simulink model "power_wind_dfig_avg"  (R2022b)
settings: Solver=ode113  StartTime=0.0  StopTime=200  RelTol=1e-3
PreLoadFcn:
  | Ts=5e-6;
InitFcn:
  | %load myModel_init;
  | Ts=5e-5;
undefined symbols (not defined in the file or in its folder): D1, D11, Delta, DiscIntNeverNeededParam, find_system
libraries: powerlib_extras x72, simulink x18, eeSinusoidalMeasurement x17, simulink_extras x12, spsThreePhaseVIMeasurementLib x11, spsControlledVoltageSourceLib x8, spsThreePhaseTransformerTwoWindingsLib x5, spsThreePhasePISectionLineLib x2, spsAsynchronousMachinepuUnitsLib x2, spsThreePhaseSeriesRLCBranchLib x2, spsThreePhaseSeriesRLCLoadLib x2, spsGroundLib x2
(part 2 of 6)

== system power_wind_dfig_avg/Wind Farm ==
  note: 9 MW Wind Farm
      | (6 x 1.5 MW)
  25 kV/ 575 V 6*1.75MVA : spsThreePhaseTransformerTwoWindingsLib/Three-Phase Transformer (Two Windings)  Winding1Connection=Delta (D11)  Winding2Connection=Yg  CoreType=Three single-phase transformers  SetSaturation=off  Hysteresis=off  DataFile='hysteresis'  SetInitialFlux=off  Measurements=None  UNITS=pu  NominalPower="[1.75e6*NoT  60]"  Winding1=[25e3 , 1e-6 0.15]  Winding2=[ 575, 1e-6 0]  Rm=500  Lm=500  L0=0.5  Saturation=[ 0,0 ; 0.0024,1.2 ; 1.0,1.52 ]  InitialFluxes=[ 0.8 , -0.8 , 0.7 ]  BreakLoop=off  DiscreteSolver=Trapezoidal iterative  DataType=off  TransfoNumber=0
  30 km line : spsThreePhasePISectionLineLib/Three-Phase PI Section Line  LConnTagsString=a|b|c  RConnTagsString=A|B|C  Length=30  Frequency=60  Resistances=[0.1153 0.413]  Inductances=[1.05e-3 3.32e-3]  Capacitances=[11.33e-009 5.01e-009]
  B25 : spsThreePhaseVIMeasurementLib/Three-Phase V-I Measurement  VoltageMeasurement=phase-to-ground  SetLabelV=off  LabelV=Vabc_B230  Vpu=on  VpuLL=off  CurrentMeasurement=yes  SetLabelI=off  LabelI=Iabc_B230  Ipu=on  Pbase=NoT*1.5e6/0.9  Vbase=25e3  OutputType=Complex  PhasorSimulation=off  PSBequivalent=0
  B575 (575 V) : spsThreePhaseVIMeasurementLib/Three-Phase V-I Measurement  VoltageMeasurement=phase-to-ground  SetLabelV=off  LabelV=Vabc_B575  Vpu=on  VpuLL=off  CurrentMeasurement=yes  SetLabelI=off  LabelI=Iabc_B575  Ipu=on  Pbase=NoT*1.5e6/0.9  Vbase=575  OutputType=Complex  PhasorSimulation=off  PSBequivalent=0
  Bus Creator : BusCreator  Inputs=5
  Bus Creator1 : BusCreator  Inputs=2
  Bus Selector1 : BusSelector  OutputSignals=Vdc_V,wr_pu (IG speed),PQ_pu.P_pu,PQ_pu.Q_pu
  Bus Selector2 : BusSelector  OutputSignals=Magnitude_sig.phiqrA,Magnitude_sig.phidrA,Magnitude_sig.iqsA,Magnitude_sig.idsA,Magnitude_sig.VqrA,Magnitude_sig.VdrA,m.Mechanical.Rotor speed (wm),m.Mechanical.Electromagnetic torque Te (pu),m.Rotor measurements.Rotor flux phir_q (pu),m.Rotor measurements.Rotor flux phir_d (pu),m.Stator measurements.Stator flux phis_q (pu),m.Stator measurements.Stator flux phis_d (pu)  OutputAsBus=on
  Constant : Constant  Value=TurOn
  Constant2 : Constant  Value=11
  Constant3 : Constant  Value=0
  DFIG Wind Turbine : Subsystem  LoadFcn=%find_system(gcs,'FollowLinks', 'on', 'LookUnderMasks', 'all');  mask(DFIG Wind Turbine){Nb_wt=NoT, ShowParameters=Generator data for 1 wind turbine, nom=[1.5e6/.9 575 1975 60], sta=[ 0.023 0.18], rot=[ 0.016 0.16], Lm=2.9, mec=[0.685 0.01 3], init=[ -0.2,0   0,0,0   0,0,0 ], Imax_grid_conv=0.8, RL_grid=[ 0.3 0.003], Vdc_nom=1150, C_DClink1=10000e-6, C_var_filter1=120e3, Pmec1=1.5e6, wind_speed_CpMax=11, wind0=11, DisplayTurbChar=off, H_WT=4.32, Ksh=1.11, D_mutual=1.5, w_wt0=1.2, torque0=0.83, Kdc=[8   400], Kgrid_side_cur_reg=[0.83 5], Kspeed=[3 0.6], Krotor_side_cur_reg=[0.6 8], Ki_QV=[0.05 20], Kp_pitch=[150], Kcompensation=[3 30], pitch_max=27, pitch_rate=0}
      mask prompts: Nb_wt "Number of wind turbines:"; ShowParameters "Display:"; nom "Nom. power, L-L volt. and freq. [Pn (VA), Vs_nom (Vrms), Vr_nom (Vrms), fn (Hz)]:"; sta "Stator [ Rs,Lls ] (p.u.):"; rot "Rotor [ Rr',Llr' ] (p.u.):"; Lm "Magnetizing inductance Lm (p.u.):"; mec "Inertia constant, friction factor, and pairs of poles [ H(s)  F(p.u.)  p ]:"; init "Initial conditions [s  th  ias  ibs  ics  phaseas phasebs phasecs]:"; Imax_grid_conv "Grid-side converter maximum current (pu of generator nominal current):"; RL_grid "Grid-side coupling inductor [ L, R] (p.u.):"; Vdc_nom "Nominal DC bus voltage (V):"; C_DClink1 "DC bus capacitor (F):"; C_var_filter1 "Line filter capacitor (Q=50) (var):"; Pmec1 "Nominal mechanical output power (W):"; wind_speed_CpMax "Wind speed at nominal speed and at Cp max (must be between 6 m/s and 30 m/s) (m/s):"; wind0 "Initial wind speed (m/s):"; DisplayTurbChar "Display wind turbine power characteristics:"; H_WT "Wind turbine inertia constant H (s):"; Ksh "Shaft spring constant refer to high-speed shaft (pu of nominal mechanical torque/rad):"; D_mutual "Shaft mutual damping (pu of nominal mechanical torque/pu dw):"; w_wt0 "Turbine initial speed (pu of nominal speed):"; torque0 "Initial output torque (pu of nominal mechanical torque):"; Kdc "DC bus voltage regulator gains [Kp Ki]:"; Kgrid_side_cur_reg "Grid-side converter current regulator gains [Kp Ki]:"; Kspeed "Speed regulator gains [Kp Ki]:"; Krotor_side_cur_reg "Rotor-side converter current regulator gains [Kp Ki]:"; Ki_QV "Q and V regulator gains [Ki_var Ki_volt]:"; Kp_pitch "Pitch controller gain [Kp]:"; Kcompensation "Pitch compensation gains [Kp Ki]:"; pitch_max "Maximum pitch angle (deg):"; pitch_rate "Maximum rate of change of pitch angle (deg/s):"
      mask help: This block implements a model of a variable speed pitch controlled wind turbine using a doubly-fed induction generator (DFIG).
      mask init: same as power_wind_dfig_avg/DFIG Wind Turbine
      mask TypeOptions ShowParameters: Generator data for 1 wind turbine | Converters data for 1 wind turbine | Turbine data for 1 wind turbine | Drive train data for 1 wind turbine | Control parameters for 1 wind turbine
      mask Callback ShowParameters:
      | BlockName=getfullname(gcb);
      | %
      | Param_Show=get_param(BlockName,'ShowParameters');
      | Param_DisplayTurbChar=get_param(BlockName,'DisplayTurbChar');
      | 
      | p_mask{3}='off';p_mask{4}='off';p_mask{5}='off';
      | p_mask{6}='off';p_mask{7}='off';p_mask{8}='off';p_mask{9}='off';
      | p_mask{10}='off';p_mask{11}='off';p_mask{12}='off';p_mask{13}='off';
      | p_mask{14}='off';p_mask{15}='off';p_mask{16}='off';p_mask{17}='off';
      | p_mask{18}='off';p_mask{19}='off';p_mask{20}='off';p_mask{21}='off';
      | p_mask{22}='off';p_mask{23}='off';p_mask{24}='off';p_mask{25}='off';
      | p_mask{26}='off';p_mask{27}='off';p_mask{28}='off';p_mask{29}='off';
      | p_mask{30}='off';p_mask{31}='off';
      | 
      | 
      | switch Param_Show
      | 	case 'Generator data for 1 wind turbine'
      | 		p_mask{3}='on';p_mask{4}='on';p_mask{5}='on'; p_mask{6}='on';
      |         p_mask{7}='on'; p_mask{8}='on';
      |     case 'Converters data for 1 wind turbine'
      | 		p_mask{9}='on';p_mask{10}='on';p_mask{11}='on';p_mask{12}='on';
      |         p_mask{13}='on';
      | 	case 'Turbine data for 1 wind turbine'
      |         p_mask{14}='on';p_mask{15}='on';p_mask{16}='on';p_mask{17}='on';
      |     case 'Drive train data for 1 wind turbine'
      |         p_mask{18}='on';p_mask{19}='on';p_mask{20}='on';p_mask{21}='on';
      |         p_mask{22}='on';
      |     case 'Control parameters for 1 wind turbine'
      |         p_mask{23}='on';p_mask{24}='on';p_mask{25}='on';
      |         p_mask{26}='on';p_mask{27}='on';p_mask{28}='on';p_mask{29}='on';
      |         p_mask{30}='on'; p_mask{31}='on';
      | end
      | 
      | ParVisible={'on','on',p_mask{3},p_mask{4},p_mask{5},p_mask{6},p_mask{7},...
      |     p_mask{8},p_mask{9},p_mask{10},p_mask{11},p_mask{12},p_mask{13},...
      |     p_mask{14},p_mask{15},p_mask{16},p_mask{17},p_mask{18},p_mask{19},...
      |     p_mask{20},p_mask{21},p_mask{22},p_mask{23},p_mask{24},p_mask{25},...
      |     p_mask{26},p_mask{27},p_mask{28},p_mask{29},p_mask{30},p_mask{31},...
      |     };
      | %
      | set_param(BlockName,'MaskVisibilities',ParVisible);
      | set_param(BlockName,'DisplayTurbChar',Param_DisplayTurbChar);
  Demux : Demux  Commented=on  Outputs=2
  From10 : From  Commented=on  GotoTag=Q_pu
      settings: CloseFcn=tagdialog Close
  From11 : From  Commented=on  GotoTag=P_pu
      settings: CloseFcn=tagdialog Close
  From3 : From  Commented=on  GotoTag=Vabc_B230
      settings: CloseFcn=tagdialog Close
  From4 : From  Commented=on  GotoTag=Iabc_B230
      settings: CloseFcn=tagdialog Close
  From6 : From  Commented=on  GotoTag=Vdc
      settings: CloseFcn=tagdialog Close
  From7 : From  Commented=on  GotoTag=wr
      settings: CloseFcn=tagdialog Close
  From8 : From  Commented=on  GotoTag=Vabc_B575
      settings: CloseFcn=tagdialog Close
  From9 : From  Commented=on  GotoTag=Iabc_B575
      settings: CloseFcn=tagdialog Close
  MW : Gain  Commented=on  Gain=NoT*1.5/0.9  SaturateOnIntegerOverflow=on  OutDataTypeStr=Inherit: Same as input  ParamDataTypeStr=Inherit: Same as input
  Manual Switch : ManualSwitch  CurrentSetting=0
  Mux : Mux  Commented=on  Inputs=2
  "Power (3ph, Instantaneous)" : spsPower3phInstantaneousLib/Power (3ph, Instantaneous)
  Product : Product  Inputs=3
  Scope : Scope  Commented=on  NumInputPorts=8
  Sine Wave Function : Sin  Amplitude=Ampl  Frequency=2*pi*Freq  Phase=0/4*pi  SampleTime=0
  Step : Step  Time=Stept  SampleTime=0
  Sum : Sum  Inputs=|+-
  Sum1 : Sum  Inputs=++|
  Terminator : Terminator
  Terminator1 : Terminator
  Three-Phase Sinusoidal Measurement (PLL) : eeSinusoidalMeasurement/Sinusoidal Measurement (PLL, Three-Phase)  Kp_LF=200  Ki_LF=2000  F0=60  Theta0=0  Ts=-1
  Three-Phase Sinusoidal Measurement (PLL)1 : eeSinusoidalMeasurement/Sinusoidal Measurement (PLL, Three-Phase)  Kp_LF=200  Ki_LF=2000  F0=60  Theta0=0  Ts=-1
  To Workspace : ToWorkspace  VariableName=windspeed  SaveFormat=Timeseries  SampleTime=-1
  wind speed m : Subsystem
  A : PMIOPort  Side=Left
  B : PMIOPort  Port=2  Side=Left
  C : PMIOPort  Port=3  Side=Left
  Macsig : Outport  VectorParamsAs1DForOutWhenUnconnected=off
  Gridsig : Outport  Port=2  VectorParamsAs1DForOutWhenUnconnected=off
  wires:
  [Vabc_B575] -> Three-Phase Sinusoidal Measurement (PLL)/1
  [Vabc_B575] -> "Power (3ph, Instantaneous)"/1
  Three-Phase Sinusoidal Measurement (PLL)/1 -> Terminator/1
  Constant3/1 -> DFIG Wind Turbine/2(Qref_pu)
  Constant2/1 -> Sum1/2
  Bus Selector1/3 -> [P_pu]  "<P_pu>"
  From3/1 -> Scope/7  "Vabc_B25 (pu)"
  Bus Creator/1 -> Gridsig/1
  Three-Phase Sinusoidal Measurement (PLL)1/2 -> Sum/2
  Demux/2 -> Scope/4  "Q (Mvar)"
  From9/1 -> Scope/2  "Iabc_B575 (pu)"
  From6/1 -> Scope/5  "Vdc (V)"
  Mux/1 -> MW/1
  Demux/1 -> Scope/3  "P (MW)"
  From4/1 -> Scope/8  "Iabc_B25 (pu)"
  [Iabc_B575] -> "Power (3ph, Instantaneous)"/2
  Bus Selector1/2 -> wind speed m/1(rotor speed), [wr]  "<wr_pu (IG speed)>"
  [Vabc_B230] -> Three-Phase Sinusoidal Measurement (PLL)1/1
  Step/1 -> Product/1
  Product/1 -> Sum1/1
  From7/1 -> Scope/6  "wr (pu)"
  Three-Phase Sinusoidal Measurement (PLL)/3 -> Bus Creator/4  "Vi"
  Bus Selector1/4 -> [Q_pu]  "<Q_pu>"
  Three-Phase Sinusoidal Measurement (PLL)1/3 -> Bus Creator/5  "Vj"
  Sine Wave Function/1 -> Product/2
  "Power (3ph, Instantaneous)"/1 -> Bus Creator/1  "SourceP"
  DFIG Wind Turbine/1(m) -> Bus Selector1/1
  From8/1 -> Scope/1  "Vabc_B575 (pu)"
  Three-Phase Sinusoidal Measurement (PLL)/2 -> Sum/1  "Thetai"
  "Power (3ph, Instantaneous)"/2 -> Bus Creator/2  "SourceQ"
  Sum/1 -> Bus Creator/3  "Thetaij"
  MW/1 -> Demux/1
  Bus Selector1/1 -> [Vdc]  "<Vdc_V>"
  From11/1 -> Mux/1
  From10/1 -> Mux/2
  Three-Phase Sinusoidal Measurement (PLL)1/1 -> Terminator1/1
  Constant/1 -> Product/3
  DFIG Wind Turbine/2(Magnitude_sig) -> Bus Creator1/1
  DFIG Wind Turbine/3(Macmeasure) -> Bus Creator1/2
  Bus Creator1/1 -> Bus Selector2/1
  Bus Selector2/1 -> Macsig/1
  B575 (575 V)/2 -> [Iabc_B575]
  B575 (575 V)/1 -> [Vabc_B575]
  B25/1 -> [Vabc_B230]
  B25/2 -> [Iabc_B230]
  wind speed m/1(wind speed) -> Manual Switch/1, To Workspace/1
  Sum1/1 -> Manual Switch/2
  Manual Switch/1 -> DFIG Wind Turbine/1("Wind (m/s) ")
  connections:
  B575 (575 V)/RConn3 -- DFIG Wind Turbine/LConn3
  B25/RConn3 -- 30 km line/LConn3
  25 kV/ 575 V 6*1.75MVA/RConn3 -- B575 (575 V)/LConn3
  B25/LConn1 -- A/RConn1
  30 km line/RConn2 -- 25 kV/ 575 V 6*1.75MVA/LConn2
  25 kV/ 575 V 6*1.75MVA/RConn2 -- B575 (575 V)/LConn2
  30 km line/RConn1 -- 25 kV/ 575 V 6*1.75MVA/LConn1
  30 km line/RConn3 -- 25 kV/ 575 V 6*1.75MVA/LConn3
  B575 (575 V)/RConn1 -- DFIG Wind Turbine/LConn1
  B25/RConn2 -- 30 km line/LConn2
  25 kV/ 575 V 6*1.75MVA/RConn1 -- B575 (575 V)/LConn1
  B575 (575 V)/RConn2 -- DFIG Wind Turbine/LConn2
  B25/RConn1 -- 30 km line/LConn1
  B25/LConn2 -- B/RConn1
  B25/LConn3 -- C/RConn1

== system power_wind_dfig_avg/info ==

== system power_wind_dfig_avg/wind speed m ==
  rotor speed : Inport
  Add : Sum
  Add1 : Sum
  Add2 : Sum
  Band-Limited White Noise : simulink/Sources/Band-Limited White Noise  Cov=[5]  Ts=0.1  seed=[34242]
  Band-Limited White Noise1 : simulink/Sources/Band-Limited White Noise  Cov=[5]  Ts=0.1  seed=[31141]
  Band-Limited White Noise2 : simulink/Sources/Band-Limited White Noise  Cov=[5]  Ts=0.1  seed=[32053]
  Cosine : simulink/Lookup Tables/Cosine  Commented=on  Formula=cos(2*pi*u)  NumDataPoints=(2^5)+1  OutputWordLength=16  InternalRulePriority=Speed
  Delay : Delay  Commented=on  DelayLength=1  InitialCondition=0
  Delay1 : Delay  Commented=on  DelayLength=1  InitialCondition=0
  Gain : Gain  Commented=on  Gain=3
  Gain1 : Gain  Commented=on  Gain=sqrt(2)
  Gain2 : Gain  Commented=on  Gain=sqrt(2)
  Gain3 : Gain  Commented=on  Gain=2*pi
  Integrator : Integrator  Commented=on  WrapState=on  WrappedStateUpperValue=2*pi  WrappedStateLowerValue=0
  Product : Product
  Product1 : Product
  Scope : Scope
  Sine : simulink/Lookup Tables/Sine  Commented=on  Formula=sin(2*pi*u)  NumDataPoints=(2^5)+1  OutputWordLength=16  InternalRulePriority=Speed
  Transfer Fcn : TransferFcn  Numerator=[4.7869 0.9904]  Denominator=[7.6823 7.3518 1]
  Transfer Fcn1 : TransferFcn  Numerator=[0.2766 0.0307]  Denominator=[0.3691 1.7722 1]
  Transfer Fcn2 : TransferFcn  Numerator=[0.2766 0.0307]  Denominator=[0.3691 1.7722 1]
  Transfer Fcn3 : TransferFcn  Numerator=[0.0182 1.3653 0.9846]  Denominator=[1.3463 3.7593 1]
  Transfer Fcn4 : TransferFcn  Numerator=[0.0182 1.3653 0.9846]  Denominator=[1.3463 3.7593 1]
  Transfer Fcn5 : TransferFcn  Numerator=[0.0182 1.3653 0.9846]  Denominator=[1.3463 3.7593 1]
  average wind speed : Constant  Value=11
  wind speed : Outport  VectorParamsAs1DForOutWhenUnconnected=off
  wires:
  average wind speed/1 -> Add/1
  Transfer Fcn/1 -> Add/2
  Delay1/1 -> Product1/1
  Gain1/1 -> Delay/1
  Transfer Fcn5/1 -> Transfer Fcn2/1
  Add2/1 -> wind speed/1, Scope/1
  Add/1 -> Add2/1
  Band-Limited White Noise2/1 -> Transfer Fcn5/1
  Delay/1 -> Product/2
  Cosine/1 -> Gain2/1
  Product/1 -> Add1/1
  Add1/1 -> Add2/2
  Gain2/1 -> Delay1/1
  Transfer Fcn3/1 -> Transfer Fcn1/1
  Band-Limited White Noise1/1 -> Transfer Fcn3/1
  Transfer Fcn2/1 -> Product1/2
  Product1/1 -> Add1/2
  Gain/1 -> Cosine/1, Sine/1
  Sine/1 -> Gain1/1
  Band-Limited White Noise/1 -> Transfer Fcn4/1
  Transfer Fcn4/1 -> Transfer Fcn/1
  Transfer Fcn1/1 -> Product/1
  Integrator/1 -> Gain/1
  rotor speed/1 -> Gain3/1
  Gain3/1 -> Integrator/1

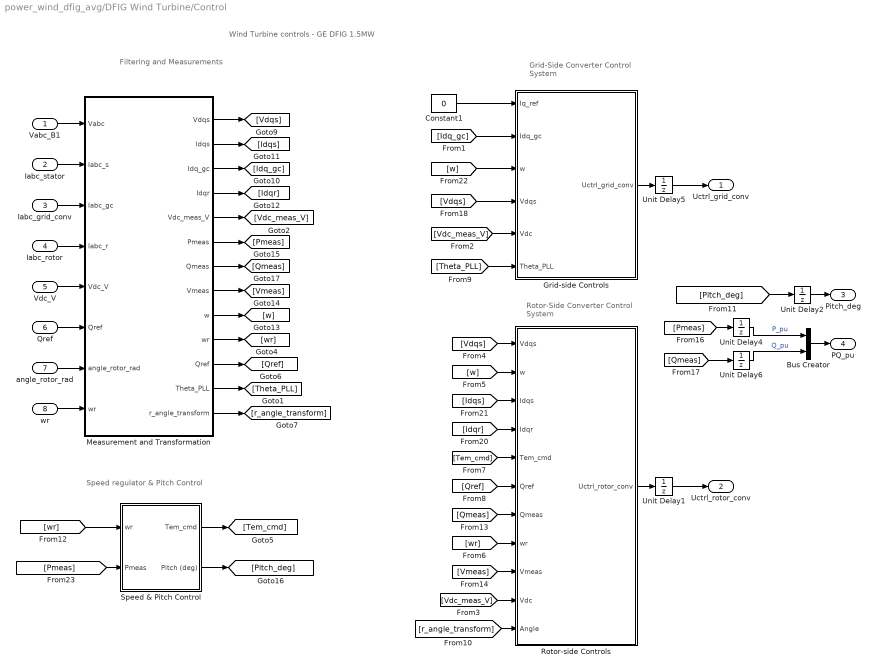
== system power_wind_dfig_avg/DFIG Wind Turbine/Control ==
  note: Speed regulator & Pitch Control
  note: Grid-Side Converter
      | Control System
  note: Rotor-Side Converter
      | Control System
  note: Filtering and
      | Measurements
  note: Wind Turbine controls - GE DFIG 1.5MW
  Vabc_B1 : Inport
  Iabc_stator : Inport  Port=2
  Iabc_grid_conv : Inport  Port=3
  Iabc_rotor : Inport  Port=4
  Vdc_V : Inport  Port=5
  Qref : Inport  Port=6
  angle_rotor_rad : Inport  Port=7
  wr : Inport  Port=8
  Bus Creator : BusCreator  Inputs=2
  Constant1 : Constant  Value=0
  Grid-side Controls : Subsystem
  Measurement and Transformation : Subsystem
  Rotor-side Controls : Subsystem
  Speed & Pitch Control : Subsystem
  Unit Delay{1..2,4..6} (5 alike) : UnitDelay  SampleTime=Ts  HasFrameUpgradeWarning=on
  Uctrl_grid_conv : Outport  VectorParamsAs1DForOutWhenUnconnected=off
  Uctrl_rotor_conv : Outport  Port=2  VectorParamsAs1DForOutWhenUnconnected=off
  Pitch_deg : Outport  Port=3  VectorParamsAs1DForOutWhenUnconnected=off
  PQ_pu : Outport  Port=4  VectorParamsAs1DForOutWhenUnconnected=off
  wires:
  Unit Delay6/1 -> Bus Creator/2  "Q_pu"
  Unit Delay4/1 -> Bus Creator/1  "P_pu"
  [Qmeas] -> Unit Delay6/1
  [Pmeas] -> Unit Delay4/1
  Bus Creator/1 -> PQ_pu/1
  Unit Delay2/1 -> Pitch_deg/1
  Unit Delay1/1 -> Uctrl_rotor_conv/1
  Unit Delay5/1 -> Uctrl_grid_conv/1
  Speed & Pitch Control/1(Tem_cmd) -> [Tem_cmd]
  Speed & Pitch Control/2(Pitch (deg)) -> [Pitch_deg]
  Rotor-side Controls/1(Uctrl_rotor_conv) -> Unit Delay1/1
  [r_angle_transform] -> Rotor-side Controls/11(Angle)
  [Vdc_meas_V] -> Rotor-side Controls/10(Vdc)
  Measurement and Transformation/13(r_angle_transform) -> [r_angle_transform]
  Grid-side Controls/1(Uctrl_grid_conv) -> Unit Delay5/1
  [Theta_PLL] -> Grid-side Controls/6(Theta_PLL)
  Measurement and Transformation/12(Theta_PLL) -> [Theta_PLL]
  [Vmeas] -> Rotor-side Controls/9(Vmeas)
  Measurement and Transformation/8(Vmeas) -> [Vmeas]
  [Qmeas] -> Rotor-side Controls/7(Qmeas)
  Measurement and Transformation/7(Qmeas) -> [Qmeas]
  Vabc_B1/1 -> Measurement and Transformation/1(Vabc)
  Iabc_grid_conv/1 -> Measurement and Transformation/3(Iabc_gc)
  Iabc_rotor/1 -> Measurement and Transformation/4(Iabc_r)
  Iabc_stator/1 -> Measurement and Transformation/2(Iabc_s)
  angle_rotor_rad/1 -> Measurement and Transformation/7(angle_rotor_rad)
  Constant1/1 -> Grid-side Controls/1(Iq_ref)
  Measurement and Transformation/1(Vdqs) -> [Vdqs]
  Measurement and Transformation/2(Idqs) -> [Idqs]
  Measurement and Transformation/3(Idq_gc) -> [Idq_gc]
  Measurement and Transformation/4(Idqr) -> [Idqr]
  Measurement and Transformation/6(Pmeas) -> [Pmeas]
  Measurement and Transformation/9(w) -> [w]
  [Idq_gc] -> Grid-side Controls/2(Idq_gc)
  [w] -> Grid-side Controls/3(w)
  [Vdqs] -> Grid-side Controls/4(Vdqs)
  [Vdc_meas_V] -> Grid-side Controls/5(Vdc)
  [Vdqs] -> Rotor-side Controls/1(Vdqs)
  [w] -> Rotor-side Controls/2(w)
  [Idqs] -> Rotor-side Controls/3(Idqs)
  [Idqr] -> Rotor-side Controls/4(Idqr)
  [Tem_cmd] -> Rotor-side Controls/5(Tem_cmd)
  [Qref] -> Rotor-side Controls/6(Qref)
  [wr] -> Speed & Pitch Control/1(wr)
  Measurement and Transformation/5(Vdc_meas_V) -> [Vdc_meas_V]
  Measurement and Transformation/10("wr ") -> [wr]
  Measurement and Transformation/11("Qref ") -> [Qref]
  Vdc_V/1 -> Measurement and Transformation/5(Vdc_V)
  Qref/1 -> Measurement and Transformation/6(Qref)
  wr/1 -> Measurement and Transformation/8(wr)
  [Pmeas] -> Speed & Pitch Control/2(Pmeas)
  [Pitch_deg] -> Unit Delay2/1
  [wr] -> Rotor-side Controls/8(wr)

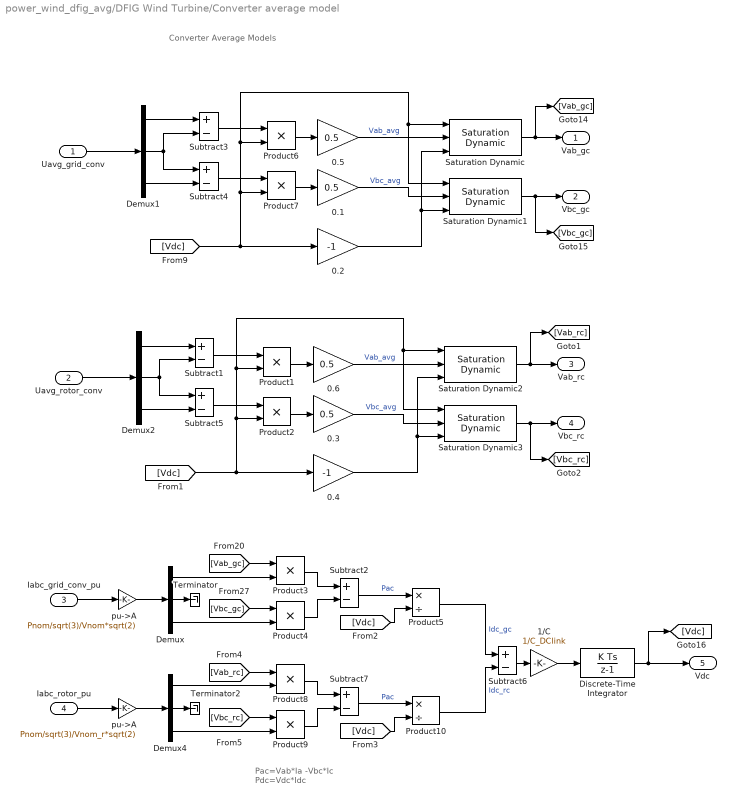
== system power_wind_dfig_avg/DFIG Wind Turbine/Converter average model ==
  note: Converter Average Models
  note: Pac=Vab*Ia -Vbc*Ic
      | Pdc=Vdc*Idc
  Uavg_grid_conv : Inport
  Uavg_rotor_conv : Inport  Port=2
  Iabc_grid_conv_pu : Inport  Port=3
  Iabc_rotor_pu : Inport  Port=4
  " pu->A" : Gain  Gain=Pnom/sqrt(3)/Vnom_r*sqrt(2)  SaturateOnIntegerOverflow=on  OutDataTypeStr=Inherit: Same as input  ParamDataTypeStr=Inherit: Same as input
  0.{1,3,5..6} (4 alike) : Gain  Gain=0.5
  0.2 : Gain  Gain=-1
  0.4 : Gain  Gain=-1
  1/C : Gain  Gain=1/C_DClink
  Demux{,1..2,4} (4 alike) : Demux  Outputs=3
  Discrete-Time Integrator : DiscreteIntegrator  InitialCondition=Vdc_nom  SampleTime=Ts  LimitOutput=on  LowerSaturationLimit=1e-6  ICPrevOutput=DiscIntNeverNeededParam  ICPrevScaledInput=DiscIntNeverNeededParam
  Product{1..4,6..9} (8 alike) : Product  RndMeth=Zero
  Product10 : Product  Inputs=*/  RndMeth=Zero
  Product5 : Product  Inputs=*/  RndMeth=Zero
  Saturation Dynamic{,1..3} (4 alike) : simulink/Discontinuities/Saturation Dynamic  OutMin=[]  OutMax=[]  OutDataTypeStr=Inherit: Same as second input  OutDataType=sfix(16)  OutScaling=2^-10  DoSatur=off
  Subtract{1..7} (7 alike) : Sum  Inputs=+-
  Terminator : Terminator
  Terminator2 : Terminator
  "pu->A " : Gain  Gain=Pnom/sqrt(3)/Vnom*sqrt(2)  SaturateOnIntegerOverflow=on  OutDataTypeStr=Inherit: Same as input  ParamDataTypeStr=Inherit: Same as input
  Vab_gc : Outport  VectorParamsAs1DForOutWhenUnconnected=off
  Vbc_gc : Outport  Port=2  VectorParamsAs1DForOutWhenUnconnected=off
  Vab_rc : Outport  Port=3  VectorParamsAs1DForOutWhenUnconnected=off
  Vbc_rc : Outport  Port=4  VectorParamsAs1DForOutWhenUnconnected=off
  Vdc : Outport  Port=5  VectorParamsAs1DForOutWhenUnconnected=off
  wires:
  " pu->A"/1 -> Demux4/1
  Demux4/2 -> Terminator2/1
  Demux4/1 -> Product8/2
  Demux4/3 -> Product9/2
  [Vdc] -> Product10/2
  [Vbc_rc] -> Product9/1
  [Vab_rc] -> Product8/1
  Product9/1 -> Subtract7/2
  Product8/1 -> Subtract7/1
  Subtract7/1 -> Product10/1  "Pac"
  Product10/1 -> Subtract6/2  "Idc_rc"
  Iabc_grid_conv_pu/1 -> "pu->A "/1
  Demux/2 -> Terminator/1
  Demux/1 -> Product3/2
  Demux/3 -> Product4/2
  Iabc_rotor_pu/1 -> " pu->A"/1
  "pu->A "/1 -> Demux/1
  Subtract6/1 -> 1/C/1
  1/C/1 -> Discrete-Time Integrator/1
  Discrete-Time Integrator/1 -> [Vdc], Vdc/1
  [Vdc] -> Product5/2
  Uavg_rotor_conv/1 -> Demux2/1
  Subtract5/1 -> Product2/1
  Subtract1/1 -> Product1/1
  Product2/1 -> 0.3/1
  Product1/1 -> 0.6/1
  Demux2/3 -> Subtract5/2
  Demux2/2 -> Subtract5/1, Subtract1/2
  Demux2/1 -> Subtract1/1
  0.6/1 -> Saturation Dynamic2/2  "Vab_avg"
  0.3/1 -> Saturation Dynamic3/2  "Vbc_avg"
  0.4/1 -> Saturation Dynamic3/3, Saturation Dynamic2/3
  Saturation Dynamic2/1 -> Vab_rc/1, [Vab_rc]
  Saturation Dynamic3/1 -> Vbc_rc/1, [Vbc_rc]
  [Vdc] -> Product2/2, Product1/2, Saturation Dynamic2/1, Saturation Dynamic3/1, 0.4/1
  Uavg_grid_conv/1 -> Demux1/1
  Subtract4/1 -> Product7/1
  Subtract3/1 -> Product6/1
  Product7/1 -> 0.1/1
  Product6/1 -> 0.5/1
  Demux1/3 -> Subtract4/2
  Demux1/2 -> Subtract3/2, Subtract4/1
  Demux1/1 -> Subtract3/1
  0.5/1 -> Saturation Dynamic/2  "Vab_avg"
  0.1/1 -> Saturation Dynamic1/2  "Vbc_avg"
  0.2/1 -> Saturation Dynamic/3, Saturation Dynamic1/3
  Saturation Dynamic/1 -> [Vab_gc], Vab_gc/1
  Saturation Dynamic1/1 -> [Vbc_gc], Vbc_gc/1
  [Vbc_gc] -> Product4/1
  [Vab_gc] -> Product3/1
  Product4/1 -> Subtract2/2
  Product3/1 -> Subtract2/1
  [Vdc] -> 0.2/1, Saturation Dynamic1/1, Saturation Dynamic/1, Product6/2, Product7/2
  Subtract2/1 -> Product5/1  "Pac"
  Product5/1 -> Subtract6/1  "Idc_gc"

== system power_wind_dfig_avg/DFIG Wind Turbine/Drive Train ==
  note: Shaft
  note: Turbine
  note: Wind turbine drive train based on a 2-masse model
  T_wt (pu) : Inport
  Generator speed (pu) : Inport  Port=2
  1_2H_WT : Gain  Gain=1/(2*H_WT)  SaturateOnIntegerOverflow=on  OutDataTypeStr=Inherit: Same as input  ParamDataTypeStr=Inherit: Same as input
  Discrete-Time Integrator : DiscreteIntegrator  InitialCondition=w_wt0  SampleTime=Ts  ICPrevOutput=DiscIntNeverNeededParam  ICPrevScaledInput=DiscIntNeverNeededParam
  Discrete-Time Integrator1 : DiscreteIntegrator  InitialCondition=torque0/Ksh  SampleTime=Ts  ICPrevOutput=DiscIntNeverNeededParam  ICPrevScaledInput=DiscIntNeverNeededParam
  Mutual damping : Gain  Gain=D_mutual  SaturateOnIntegerOverflow=on  OutDataTypeStr=Inherit: Same as input  ParamDataTypeStr=Inherit: Same as input
  Stiffness : Gain  Gain=Ksh  SaturateOnIntegerOverflow=on  OutDataTypeStr=Inherit: Same as input  ParamDataTypeStr=Inherit: Same as input
  Sum : Sum  Inputs=+-  InputSameDT=on  SaturateOnIntegerOverflow=on  OutDataTypeStr=Inherit: Same as first input
  Sum1 : Sum  Inputs=+-  InputSameDT=on  SaturateOnIntegerOverflow=on  OutDataTypeStr=Inherit: Same as first input
  Sum2 : Sum  InputSameDT=on  SaturateOnIntegerOverflow=on  OutDataTypeStr=Inherit: Same as first input
  wbase : Gain  Gain=wbase  SaturateOnIntegerOverflow=on  OutDataTypeStr=Inherit: Same as input  ParamDataTypeStr=Inherit: Same as input
  W_wt (pu) : Outport  VectorParamsAs1DForOutWhenUnconnected=off
  T_shaft (pu) : Outport  Port=2  VectorParamsAs1DForOutWhenUnconnected=off
  wires:
  wbase/1 -> Discrete-Time Integrator1/1
  Discrete-Time Integrator1/1 -> Stiffness/1
  Stiffness/1 -> Sum2/1
  Sum/1 -> 1_2H_WT/1
  1_2H_WT/1 -> Discrete-Time Integrator/1
  Discrete-Time Integrator/1 -> Sum1/1, W_wt (pu)/1
  Generator speed (pu)/1 -> Sum1/2
  Sum1/1 -> wbase/1, Mutual damping/1
  Mutual damping/1 -> Sum2/2
  Sum2/1 -> Sum/2, T_shaft (pu)/1
  T_wt (pu)/1 -> Sum/1

== system power_wind_dfig_avg/DFIG Wind Turbine/Wind Turbine ==
  W_wt (pu) : Inport
  Pitch angle (deg) : Inport  Port=2
  Wind speed (m/s) : Inport  Port=3
  ->pu : Gain  Gain=1/Prated
  Avoid div. by zero : Saturate  UpperLimit=inf  LowerLimit=eps
  "Avoid div. by zero " : Saturate  UpperLimit=inf  LowerLimit=eps
  Fcn1 : Fcn  Expr=K1*u[2]/u[1]
  Fcn2 : Fcn  Expr=c1*(c6*u[1] + (-c4 - c3*(2.5 + u[2]) + c2*(1/(u[1] + c7*(2.5 + u[2])) -c8/(1 + (2.5 + u[2])^3)))/exp(c5*(1/(u[1] + c7*(2.5 + u[2])) - c8/(1 + (2.5 + u[2])^3))))
  "K2*Cp*wind^3 " : Fcn  Expr=K2*u[1]^3*u[2]
  Mux : Mux  Inputs=2
  Mux1 : Mux  Inputs=2
  Mux2 : Mux  Inputs=2
  Product2 : Product  Inputs=*/  InputSameDT=on  SaturateOnIntegerOverflow=on  OutDataTypeStr=Inherit: Same as first input
  Tt (pu) : Outport  VectorParamsAs1DForOutWhenUnconnected=off
  wires:
  "K2*Cp*wind^3 "/1 -> ->pu/1
  "Avoid div. by zero "/1 -> Product2/2, Mux/2
  Avoid div. by zero/1 -> Mux/1, Mux2/1
  W_wt (pu)/1 -> "Avoid div. by zero "/1
  Pitch angle (deg)/1 -> Mux1/2
  Mux2/1 -> "K2*Cp*wind^3 "/1
  Fcn2/1 -> Mux2/2  "Cp"
  Mux/1 -> Fcn1/1
  Mux1/1 -> Fcn2/1
  Fcn1/1 -> Mux1/1  "lambda"
  Wind speed (m/s)/1 -> Avoid div. by zero/1
  Product2/1 -> Tt (pu)/1
  ->pu/1 -> Product2/1  "power_pu"

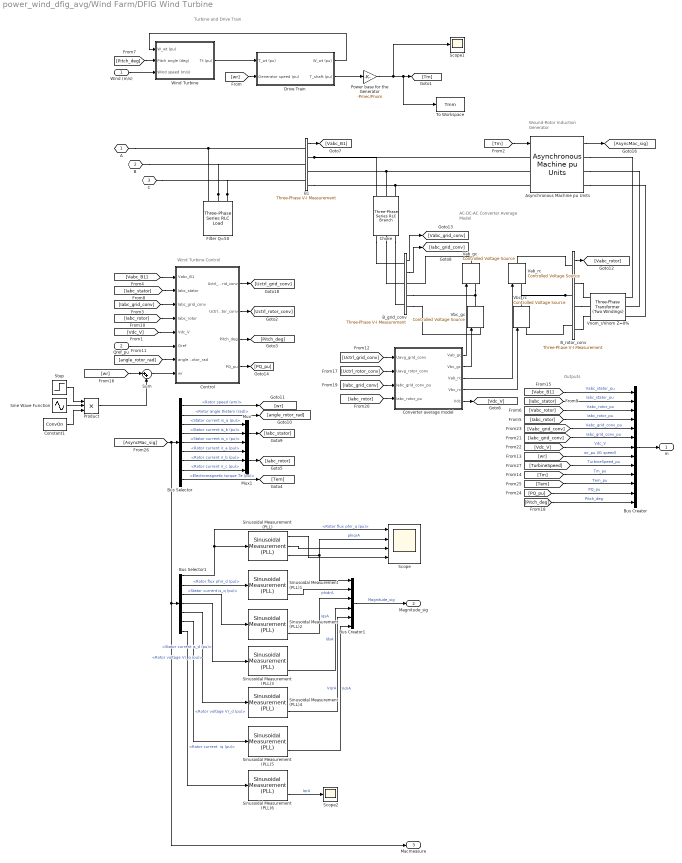
== system power_wind_dfig_avg/Wind Farm/DFIG Wind Turbine ==
  note: Turbine and Drive Train
  note: Wind Turbine Control
  note: Wound-Rotor
      | Induction Generator
  note: AC-DC-AC Converter
      | Average Model
  note: Outputs
  "Wind (m/s) " : Inport
  Qref_pu : Inport  Port=2
  Asynchronous Machine pu Units : spsAsynchronousMachinepuUnitsLib/Asynchronous Machine pu Units  RotorType=Wound  PresetModel=No  MechanicalLoad=Torque Tm  ShowDetailedParameters=on  ReferenceFrame=Rotor  Units=pu  MeasurementBus=off  NominalParameters=[ Pnom Vnom Fnom ]  VoltageRatio=1  Stator=[ Rs Lls]  Rotor=[ Rr Llr]  Cage1=[0.01909 0.0397]  Cage2=[0.01909 0.0397]  Lm=Lm  Mechanical=[H F p]  PolePairs=3  InitialConditions=init  SimulateSaturation=off  Saturation="[0.212,0.4201,0.8125,1.0979,1.4799,2.2457,3.2586,4.5763,6.4763 ;   0.5,0.7,0.9,1,1.1,1.2 ,1.3,1.4,1.5]"  LoadFlowParameters=0  TsPowergui=0  TsBlock=-1  IterativeModel=Trapezoidal non iterative  IterativeDiscreteModel=Trapezoidal non iterative  Pmec=0
      settings: LibrarySourceBlock=|
      | sps_lib/Electrical Machines/Asynchronous Machine
      | pu Units
  B1 : spsThreePhaseVIMeasurementLib/Three-Phase V-I Measurement  VoltageMeasurement=phase-to-ground  SetLabelV=off  LabelV=Vabc  Vpu=on  VpuLL=off  CurrentMeasurement=no  SetLabelI=on  LabelI=Iabc_B1  Ipu=on  Pbase=Pnom  Vbase=Vnom  OutputType=Complex  PhasorSimulation=off  PSBequivalent=0
  B_grid_conv : spsThreePhaseVIMeasurementLib/Three-Phase V-I Measurement  VoltageMeasurement=phase-to-ground  SetLabelV=off  LabelV=Vabc_B1  Vpu=on  VpuLL=off  CurrentMeasurement=yes  SetLabelI=off  LabelI=Iabc  Ipu=on  Pbase=Pnom  Vbase=Vnom  OutputType=Complex  PhasorSimulation=off  PSBequivalent=0
  B_rotor_conv : spsThreePhaseVIMeasurementLib/Three-Phase V-I Measurement  VoltageMeasurement=phase-to-phase  SetLabelV=off  LabelV=Vabc_B1  Vpu=on  VpuLL=off  CurrentMeasurement=no  SetLabelI=off  LabelI=Iabc  Ipu=on  Pbase=Pnom  Vbase=Vnom_r  OutputType=Complex  PhasorSimulation=off  PSBequivalent=0
  Bus Creator : BusCreator  Inputs=13
  Bus Creator1 : BusCreator  Inputs=6
  Bus Selector : BusSelector  OutputSignals=Mechanical.Rotor speed (wm),Mechanical.Rotor angle thetam (rad),Stator measurements.Stator current is_a (pu),Stator measurements.Stator current is_b (pu),Stator measurements.Stator current is_c (pu),Rotor measurements.Rotor current ir_a (pu),Rotor measurements.Rotor current ir_b (pu),Rotor measurements.Rotor current ir_c (pu),Mechanical.Electromagnetic torque Te (pu)
  Bus Selector1 : BusSelector  OutputSignals="Rotor measurements.Rotor flux phir_q (pu),Rotor measurements.Rotor flux phir_d (pu),Stator measurements.Stator current is_q (pu),Stator measurements.Stator current is_d (pu),Rotor measurements.Rotor voltage Vr_q (pu),Rotor measurements.Rotor voltage Vr_d (pu),Rotor measurements.Rotor current  iq (pu)"
  "Choke " : spsThreePhaseSeriesRLCBranchLib/Three-Phase Series RLC Branch  LConnTagsString=A|B|C  RConnTagsString=A|B|C  BranchType=RL  Resistance=R_RL*Vnom^2/Pnom  Inductance=L_RL*Vnom^2/Pnom/(2*pi*Fnom)  Capacitance=[]  Measurements=None
  Constant1 : Constant  Value=ConvOn
  Control : Subsystem
  Converter average model : Subsystem
  Drive Train : Subsystem  mask(Wind Turbine shaft){H_WT=H_WT, Ksh=Ksh, D_mutual=D_mutual, wbase=2*pi*Fnom/p, w_wt0=w_wt0, torque0=torque0, Ts=Ts}
      mask prompts: H_WT "Wind turbine inertia constant H (s):"; Ksh "Shaft spring constant (pu of nominal mechanical torque/rad):"; D_mutual "Shaft mutual damping (pu of nominal mechanical torque/pu dw):"; wbase "Shaft base speed (rad/s):"; w_wt0 "Turbine initial speed (pu of base speed):"; torque0 "Initial output torque (pu of nominal mechanical torque):"; Ts "Sample time (s):"
      mask help:
      | This block implements a wind turbine drive train model. All shaft parameters are referred to high-speed shaft (generator shaft).
      |
      | The first input is the wind turbine torque in per unit (pu) based on the nominal power of the turbine and the base speed of the generator. The second input is the generator speed in pu based on the base speed of the generator.
      |
      | The outputs are:
      | 1- the transmitted torque of the shaft in pu based on the nominal power of the turbine and the base speed of the generator.
      | 2- the wind turbine speed in pu of the base speed of the generator.
  Filter Q=50 : spsThreePhaseSeriesRLCLoadLib/Three-Phase Series RLC Load  LConnTagsString=A|B|C  Configuration=Y (grounded)  NominalVoltage=Vnom  Vabc=[1e3 1e3 1e3]  Vabcp=[1e3 1e3 1e3]  NominalFrequency=Fnom  UnbalancedPower=off  ActivePower=C_var_filter/Q_filter  InductivePower=0  CapacitivePower=C_var_filter  Pabc=[10e3 9e3 11e3]  QLabc=[100 90 110]  QCabc=[100 90 110]  Pabcp=[10e3 9e3 11e3]  QLabcp=[100 90 110]  QCabcp=[100 90 110]  Measurements=None  LoadType=constant Z
  Mux : Mux  Inputs=3
  Mux1 : Mux  Inputs=3
  Power base for the Generator : Gain  Gain=-Pmec/Pnom  SaturateOnIntegerOverflow=on  OutDataTypeStr=Inherit: Same as input  ParamDataTypeStr=Inherit: Same as input
  Product : Product  Inputs=3
  Scope : Scope  NumInputPorts=4
  Scope1 : Scope
  Scope2 : Scope
  Sine Wave Function : Sin  Amplitude=Ampl  Frequency=2*pi*Freq  Phase=0/4*pi  SampleTime=0
  Sinusoidal Measurement (PLL) : eeSinusoidalMeasurement/Sinusoidal Measurement (PLL)  Ki_PD=600  Kp_LF=10000  Ki_LF=10000  F0=21  Theta0=0  Mag0=0  Ts=-1
  Sinusoidal Measurement (PLL)1 : eeSinusoidalMeasurement/Sinusoidal Measurement (PLL)  Ki_PD=200  Kp_LF=200  Ki_LF=7500  F0=0.5  Theta0=0  Mag0=1  Ts=-1
  Sinusoidal Measurement (PLL){2..6} (5 alike) : eeSinusoidalMeasurement/Sinusoidal Measurement (PLL)  Ki_PD=200  Kp_LF=200  Ki_LF=2000  F0=10.8  Theta0=0  Mag0=1  Ts=-1
  Step : Step  Time=Stept  SampleTime=0
  Sum : Sum  Inputs=|++
  To Workspace : ToWorkspace  VariableName=Tmm  SaveFormat=Timeseries  SampleTime=-1
  Vab_gc : spsControlledVoltageSourceLib/Controlled Voltage Source  Initialize=on  Source_Type=AC  Amplitude=0  Phase=0  Frequency=0  Measurements=None
  Vab_rc : spsControlledVoltageSourceLib/Controlled Voltage Source  Initialize=on  Source_Type=AC  Amplitude=0  Phase=0  Frequency=0  Measurements=None
  Vbc_gc : spsControlledVoltageSourceLib/Controlled Voltage Source  Initialize=on  Source_Type=AC  Amplitude=0  Phase=0  Frequency=0  Measurements=None
  Vbc_rc : spsControlledVoltageSourceLib/Controlled Voltage Source  Initialize=on  Source_Type=AC  Amplitude=0  Phase=0  Frequency=0  Measurements=None
  Vnom_r/Vnom Z=0% : spsThreePhaseTransformerTwoWindingsLib/Three-Phase Transformer (Two Windings)  Winding1Connection=Y  Winding2Connection=Y  CoreType=Three single-phase transformers  SetSaturation=off  Hysteresis=off  DataFile='hysteresis'  SetInitialFlux=off  Measurements=None  UNITS=pu  NominalPower=[ Pnom , Fnom ]  Winding1=[ Vnom_r , 0, 0]  Winding2=[ Vnom , 0, 0]  Rm=500  Lm=inf  L0=0.5  Saturation=[ 0,0 ; 0.0024,1.2 ; 1.0,1.52 ]  InitialFluxes=[ 0.8 , -0.8 , 0.7 ]  BreakLoop=off  DiscreteSolver=Trapezoidal iterative  DataType=off  TransfoNumber=0
  Wind Turbine : Subsystem  mask(Wind Turbine){Prated=Pmec, c1_c8=c1_c8, K1_K2=K1_K2, wind0=wind0, Ts=Ts}
      mask prompts: Prated "Nominal mechanical output power (W):"; c1_c8 "Coefficients [c1 ... c8]"; K1_K2 "Parameters [K1 K2]"; wind0 "Initial wind speed (m/s):"; Ts "Sample time (s):"
      mask help:
      | This block implements a generic wind turbine models.
      |
      | The first input is the turbine speed in per unit of the generator base speed. For a synchronous or asynchronous generator, the base speed is the synchronous speed. For a permanent-magnet generator, the base speed is defined as the speed producing nominal voltage at  no load. The second input is the blade pitch angle in degrees. The third input is the wind speed in m/s.
      |
      | The output is the torque applied to the drive train in per unit based on the nominal power of the turbine and the base speed of the generator.
      mask init:
      | c1 = c1_c8(1);
      | c2 = c1_c8(2);
      | c3 = c1_c8(3);
      | c4 = c1_c8(4);
      | c5 = c1_c8(5);
      | c6 = c1_c8(6);
      | c7 = c1_c8(7);;
      | c8 = c1_c8(8);
      | 
      | K1=K1_K2(1);
      | K2=K1_K2(2);
      settings: OpenFcn=power_openblockproxy();
      mask Display: disp('');
  A : PMIOPort  Tag=PMCPort  Side=Left
  B : PMIOPort  Tag=PMCPort  Port=2  Side=Left
  C : PMIOPort  Tag=PMCPort  Port=3  Side=Left
  m : Outport  VectorParamsAs1DForOutWhenUnconnected=off
  Magnitude_sig : Outport  Port=2  VectorParamsAs1DForOutWhenUnconnected=off
  Macmeasure : Outport  Port=3  VectorParamsAs1DForOutWhenUnconnected=off
  wires:
  [Pitch_deg] -> Bus Creator/13  "Pitch_deg"
  [PQ_pu] -> Bus Creator/12  "PQ_pu"
  Control/4(PQ_pu) -> [PQ_pu]
  [Tem] -> Bus Creator/11  "Tem_pu"
  [Tm] -> Bus Creator/10  "Tm_pu"
  [TurbineSpeed] -> Bus Creator/9  "TurbineSpeed_pu"
  [Vdc_V] -> Bus Creator/7  "Vdc_V"
  [Iabc_grid_conv] -> Bus Creator/6  "Iabc_grid_conv_pu"
  [Vabc_grid_conv] -> Bus Creator/5  "Vabc_grid_conv_pu"
  [Iabc_rotor] -> Bus Creator/4  "Iabc_rotor_pu"
  [Vabc_rotor] -> Bus Creator/3  "Vabc_rotor_pu"
  [Iabc_stator] -> Bus Creator/2  "Iabc_stator_pu"
  [Vabc_B1] -> Bus Creator/1  "Vabc_stator_pu"
  Asynchronous Machine pu Units/1 -> [AsyncMac_sig]
  Converter average model/5(Vdc) -> [Vdc_V]
  Converter average model/4(Vbc_rc) -> Vbc_rc/1
  Converter average model/3(Vab_rc) -> Vab_rc/1
  Converter average model/2(Vbc_gc) -> Vbc_gc/1
  Converter average model/1(Vab_gc) -> Vab_gc/1
  [Iabc_rotor] -> Converter average model/4(Iabc_rotor_pu)
  [Pitch_deg] -> Wind Turbine/2(Pitch angle (deg))
  Drive Train/1(W_wt (pu)) -> Wind Turbine/1(W_wt (pu))
  "Wind (m/s) "/1 -> Wind Turbine/3(Wind speed (m/s))
  Power base for the Generator/1 -> Scope1/1, To Workspace/1, [Tm]
  Drive Train/2(T_shaft (pu)) -> Power base for the Generator/1
  [wr] -> Drive Train/2(Generator speed (pu))
  Wind Turbine/1(Tt (pu)) -> Drive Train/1(T_wt (pu))
  Qref_pu/1 -> Control/6(Qref)
  Bus Selector/9 -> [Tem]  "<Electromagnetic torque Te (pu)>"
  Bus Selector/1 -> [wr]  "<Rotor speed (wm)>"
  Bus Creator/1 -> m/1
  B_rotor_conv/1 -> [Vabc_rotor]
  B1/1 -> [Vabc_B1]
  [Vabc_B1] -> Control/1(Vabc_B1)
  [Iabc_grid_conv] -> Control/3(Iabc_grid_conv)
  [Iabc_rotor] -> Control/4(Iabc_rotor)
  [angle_rotor_rad] -> Control/7(angle_rotor_rad)
  Mux1/1 -> [Iabc_rotor]
  Mux/1 -> [Iabc_stator]
  [Vdc_V] -> Control/5(Vdc_V)
  Control/3(Pitch_deg) -> [Pitch_deg]
  [Iabc_stator] -> Control/2(Iabc_stator)
  Bus Selector/8 -> Mux1/3  "<Rotor current ir_c (pu)>"
  Bus Selector/7 -> Mux1/2  "<Rotor current ir_b (pu)>"
  Bus Selector/6 -> Mux1/1  "<Rotor current ir_a (pu)>"
  Bus Selector/5 -> Mux/3  "<Stator current is_c (pu)>"
  Bus Selector/4 -> Mux/2  "<Stator current is_b (pu)>"
  Bus Selector/3 -> Mux/1  "<Stator current is_a (pu)>"
  Bus Selector/2 -> [angle_rotor_rad]  "<Rotor angle thetam (rad)>"
  B_grid_conv/2 -> [Iabc_grid_conv]
  B_grid_conv/1 -> [Vabc_grid_conv]
  Control/1(Uctrl_grid_conv) -> [Uctrl_grid_conv]
  Control/2(Uctrl_rotor_conv) -> [Uctrl_rotor_conv]
  [AsyncMac_sig] -> Macmeasure/1, Bus Selector1/1, Bus Selector/1
  [wr] -> Bus Creator/8  "wr_pu (IG speed)"
  [Tm] -> Asynchronous Machine pu Units/1
  Bus Creator1/1 -> Magnitude_sig/1  "Magnitude_sig"
  Bus Selector1/1 -> Scope/1, Sinusoidal Measurement (PLL)/1  "<Rotor flux phir_q (pu)>"
  Bus Selector1/2 -> Sinusoidal Measurement (PLL)1/1  "<Rotor flux phir_d (pu)>"
  Bus Selector1/3 -> Sinusoidal Measurement (PLL)2/1  "<Stator current is_q (pu)>"
  Bus Selector1/4 -> Sinusoidal Measurement (PLL)3/1  "<Stator current is_d (pu)>"
  Sinusoidal Measurement (PLL)/3 -> Bus Creator1/1, Scope/2  "phiqrA"
  Sinusoidal Measurement (PLL)1/3 -> Bus Creator1/2  "phidrA"
  Sinusoidal Measurement (PLL)2/3 -> Bus Creator1/3  "iqsA"
  Sinusoidal Measurement (PLL)3/3 -> Bus Creator1/4  "idsA"
  Sinusoidal Measurement (PLL)/2 -> Scope/3
  [wr] -> Sum/1
  Sum/1 -> Control/8(wr)
  Product/1 -> Sum/2
  Sine Wave Function/1 -> Product/2
  Step/1 -> Product/1
  [Uctrl_rotor_conv] -> Converter average model/2(Uavg_rotor_conv)
  [Iabc_grid_conv] -> Converter average model/3(Iabc_grid_conv_pu)
  [Uctrl_grid_conv] -> Converter average model/1(Uavg_grid_conv)
  Bus Selector1/5 -> Sinusoidal Measurement (PLL)4/1  "<Rotor voltage Vr_q (pu)>"
  Bus Selector1/6 -> Sinusoidal Measurement (PLL)5/1  "<Rotor voltage Vr_d (pu)>"
  Sinusoidal Measurement (PLL)4/3 -> Bus Creator1/5  "VqrA"
  Sinusoidal Measurement (PLL)5/3 -> Bus Creator1/6  "VdrA"
  Constant1/1 -> Product/3
  Bus Selector1/7 -> Sinusoidal Measurement (PLL)6/1  "<Rotor current  iq (pu)>"
  Sinusoidal Measurement (PLL)6/3 -> Scope2/1  "IqrA"
  Sinusoidal Measurement (PLL)/1 -> Scope/4
  connections:
  Filter Q=50/LConn3 -- B1/LConn3 -- C/RConn1
  Filter Q=50/LConn2 -- B1/LConn2 -- B/RConn1
  Filter Q=50/LConn1 -- B1/LConn1 -- A/RConn1
  Vbc_rc/LConn1 -- B_rotor_conv/LConn3
  Vab_rc/RConn1 -- B_rotor_conv/LConn1
  B_rotor_conv/LConn2 -- Vab_rc/LConn1 -- Vbc_rc/RConn1
  B_grid_conv/RConn3 -- Vbc_gc/LConn1
  Vab_gc/RConn1 -- B_grid_conv/RConn1
  B_grid_conv/RConn2 -- Vbc_gc/RConn1 -- Vab_gc/LConn1
  B_rotor_conv/RConn3 -- Vnom_r/Vnom Z=0%/LConn3
  B_rotor_conv/RConn2 -- Vnom_r/Vnom Z=0%/LConn2
  B_rotor_conv/RConn1 -- Vnom_r/Vnom Z=0%/LConn1
  B1/RConn3 -- "Choke "/LConn3 -- Asynchronous Machine pu Units/LConn3
  Asynchronous Machine pu Units/RConn3 -- Vnom_r/Vnom Z=0%/RConn3
  Asynchronous Machine pu Units/RConn1 -- Vnom_r/Vnom Z=0%/RConn1
  Asynchronous Machine pu Units/RConn2 -- Vnom_r/Vnom Z=0%/RConn2
  "Choke "/RConn3 -- B_grid_conv/LConn3
  "Choke "/RConn2 -- B_grid_conv/LConn2
  "Choke "/RConn1 -- B_grid_conv/LConn1
  B1/RConn1 -- Asynchronous Machine pu Units/LConn1 -- "Choke "/LConn1
  Asynchronous Machine pu Units/LConn2 -- B1/RConn2 -- "Choke "/LConn2

== system power_wind_dfig_avg/Wind Farm/wind speed m ==
  rotor speed : Inport
  Add : Sum
  Add1 : Sum
  Add2 : Sum
  Band-Limited White Noise : simulink/Sources/Band-Limited White Noise  Cov=[1]  Ts=0.1  seed=[54621]
  Band-Limited White Noise1 : simulink/Sources/Band-Limited White Noise  Cov=[1]  Ts=0.1  seed=[11750]
  Band-Limited White Noise2 : simulink/Sources/Band-Limited White Noise  Cov=[1]  Ts=0.1  seed=[59752]
  Cosine : simulink/Lookup Tables/Cosine  Formula=cos(2*pi*u)  NumDataPoints=(2^5)+1  OutputWordLength=16  InternalRulePriority=Speed
  Delay : Delay  DelayLength=1  InitialCondition=0
  Delay1 : Delay  DelayLength=1  InitialCondition=0
  Gain : Gain  Gain=3
  Gain1 : Gain  Gain=sqrt(2)
  Gain2 : Gain  Gain=sqrt(2)
  Gain3 : Gain  Gain=2*pi*1/3
  Integrator : Integrator  WrapState=on  WrappedStateUpperValue=2*pi  WrappedStateLowerValue=0
  Product : Product
  Product1 : Product
  Scope : Scope
  Sine : simulink/Lookup Tables/Sine  Formula=sin(2*pi*u)  NumDataPoints=(2^5)+1  OutputWordLength=16  InternalRulePriority=Speed
  Transfer Fcn : TransferFcn  Numerator=[4.7869 0.9904]  Denominator=[7.6823 7.3518 1]
  Transfer Fcn1 : TransferFcn  Numerator=[0.2766 0.0307]  Denominator=[0.3691 1.7722 1]
  Transfer Fcn2 : TransferFcn  Numerator=[0.2766 0.0307]  Denominator=[0.3691 1.7722 1]
  Transfer Fcn3 : TransferFcn  Numerator=[0.0182 1.3653 0.9846]  Denominator=[1.3463 3.7593 1]
  Transfer Fcn4 : TransferFcn  Numerator=[0.0182 1.3653 0.9846]  Denominator=[1.3463 3.7593 1]
  Transfer Fcn5 : TransferFcn  Numerator=[0.0182 1.3653 0.9846]  Denominator=[1.3463 3.7593 1]
  average wind speed : Constant  Value=11
  wind speed : Outport  VectorParamsAs1DForOutWhenUnconnected=off
  wires:
  average wind speed/1 -> Add/1
  Transfer Fcn/1 -> Add/2
  Delay1/1 -> Product1/1
  Gain1/1 -> Delay/1
  Transfer Fcn5/1 -> Transfer Fcn2/1
  Add2/1 -> wind speed/1, Scope/1
  Add/1 -> Add2/1
  Band-Limited White Noise2/1 -> Transfer Fcn5/1
  Delay/1 -> Product/2
  Cosine/1 -> Gain2/1
  Product/1 -> Add1/1
  Add1/1 -> Add2/2
  Gain2/1 -> Delay1/1
  Transfer Fcn3/1 -> Transfer Fcn1/1
  Band-Limited White Noise1/1 -> Transfer Fcn3/1
  Transfer Fcn2/1 -> Product1/2
  Product1/1 -> Add1/2
  Gain/1 -> Cosine/1, Sine/1
  Sine/1 -> Gain1/1
  Band-Limited White Noise/1 -> Transfer Fcn4/1
  Transfer Fcn4/1 -> Transfer Fcn/1
  Transfer Fcn1/1 -> Product/1
  Integrator/1 -> Gain/1
  rotor speed/1 -> Gain3/1
  Gain3/1 -> Integrator/1

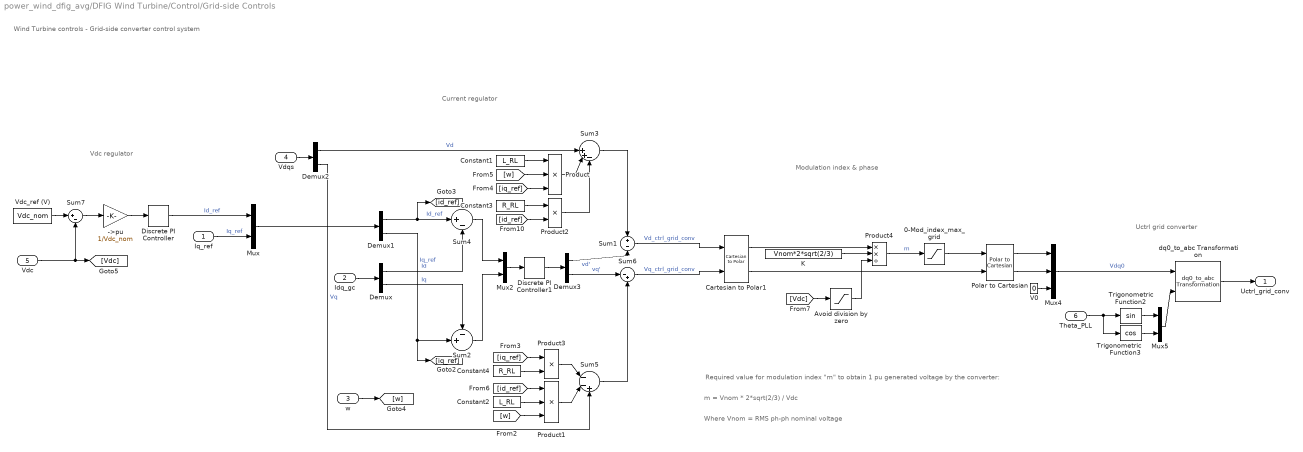
== system power_wind_dfig_avg/DFIG Wind Turbine/Control/Grid-side Controls ==
  note: Uctrl grid converter
  note: Modulation index & phase
  note: Current regulator
  note: Vdc regulator
  note: Required value for modulation index "m" to obtain 1 pu generated voltage by the converter:
  note: m = Vnom * 2*sqrt(2/3) / Vdc
  note: Where Vnom = RMS ph-ph nominal voltage
  note: Wind Turbine controls - Grid-side converter control system
  Iq_ref : Inport
  Idq_gc : Inport  Port=2
  w : Inport  Port=3
  Vdqs : Inport  Port=4
  Vdc : Inport  Port=5
  Theta_PLL : Inport  Port=6
  ->pu : Gain  Gain=1/Vdc_nom
  0-Mod_index_max_grid : Saturate  UpperLimit=Mod_index_max_grid  LowerLimit=0
  Avoid division by zero : Saturate  UpperLimit=inf  LowerLimit=1e-6
  Cartesian to Polar1 : simulink_extras/Transformations/Cartesian to Polar
  Constant1 : Constant  Value=L_RL
  Constant2 : Constant  Value=L_RL
  Constant3 : Constant  Value=R_RL
  Constant4 : Constant  Value=R_RL
  Demux{,1..3} (4 alike) : Demux  Outputs=2
      settings: DisplayOption=none
  Discrete PI Controller : powerlib_extras/Discrete  Control Blocks/Discrete PI Controller  Kp=Kp_dc  Ki=Ki_dc  Par_Limits=[1 -1]*Imax_grid_conv  Init=0  Ts=Ts
  Discrete PI Controller1 : powerlib_extras/Discrete  Control Blocks/Discrete PI Controller  Kp=Kp_grid_side_cur_reg  Ki=Ki_grid_side_cur_reg  Par_Limits=[1.0 -1.0] *Lim_grid_side_cur_reg  Init=0  Ts=Ts
  K : Constant  Value=Vnom*2*sqrt(2/3)
  Mux : Mux  Inputs=2
  Mux2 : Mux  Inputs=2
  Mux4 : Mux  Inputs=3
  Mux5 : Mux  Inputs=2
  Polar to Cartesian : simulink_extras/Transformations/Polar to Cartesian
  Product : Product  Inputs=3  InputSameDT=on  SaturateOnIntegerOverflow=on  OutDataTypeStr=Inherit: Same as first input
  Product1 : Product  Inputs=3  InputSameDT=on  SaturateOnIntegerOverflow=on  OutDataTypeStr=Inherit: Same as first input
  Product2 : Product  InputSameDT=on  SaturateOnIntegerOverflow=on  OutDataTypeStr=Inherit: Same as first input
  Product3 : Product  InputSameDT=on  SaturateOnIntegerOverflow=on  OutDataTypeStr=Inherit: Same as first input
  Product4 : Product  Inputs=**/  InputSameDT=on  SaturateOnIntegerOverflow=on  OutDataTypeStr=Inherit: Same as first input
  Sum1 : Sum  Inputs=+-  InputSameDT=on  SaturateOnIntegerOverflow=on  OutDataTypeStr=Inherit: Same as first input
  Sum2 : Sum  Inputs=-+|  InputSameDT=on  SaturateOnIntegerOverflow=on  OutDataTypeStr=Inherit: Same as first input
  Sum3 : Sum  Inputs=||++-  InputSameDT=on  SaturateOnIntegerOverflow=on  OutDataTypeStr=Inherit: Same as first input
  Sum4 : Sum  Inputs=|+-  InputSameDT=on  SaturateOnIntegerOverflow=on  OutDataTypeStr=Inherit: Same as first input
  Sum5 : Sum  Inputs=|--+  InputSameDT=on  SaturateOnIntegerOverflow=on  OutDataTypeStr=Inherit: Same as first input
  Sum6 : Sum  Inputs=|-+  InputSameDT=on  SaturateOnIntegerOverflow=on  OutDataTypeStr=Inherit: Same as first input
  Sum7 : Sum  Inputs=|+-  InputSameDT=on  SaturateOnIntegerOverflow=on  OutDataTypeStr=Inherit: Same as first input
  Trigonometric Function2 : Trigonometry
  Trigonometric Function3 : Trigonometry  Operator=cos
  V0 : Constant  Value=0
  Vdc_ref (V) : Constant  Value=Vdc_nom
  dq0_to_abc Transformation : powerlib_extras/Measurements/dq0_to_abc Transformation
  Uctrl_grid_conv : Outport  VectorParamsAs1DForOutWhenUnconnected=off
  wires:
  Sum6/1 -> Cartesian to Polar1/2  "Vq_ctrl_grid_conv"
  Sum1/1 -> Cartesian to Polar1/1  "Vd_ctrl_grid_conv"
  dq0_to_abc Transformation/1 -> Uctrl_grid_conv/1
  Theta_PLL/1 -> Trigonometric Function2/1, Trigonometric Function3/1
  Mux4/1 -> dq0_to_abc Transformation/1  "Vdq0"
  Polar to Cartesian/2 -> Mux4/2
  Polar to Cartesian/1 -> Mux4/1
  V0/1 -> Mux4/3
  Trigonometric Function3/1 -> Mux5/2
  Trigonometric Function2/1 -> Mux5/1
  Mux5/1 -> dq0_to_abc Transformation/2
  [Vdc] -> Avoid division by zero/1
  Product4/1 -> 0-Mod_index_max_grid/1  "m"
  K/1 -> Product4/2
  Avoid division by zero/1 -> Product4/3
  Cartesian to Polar1/1 -> Product4/1
  0-Mod_index_max_grid/1 -> Polar to Cartesian/1
  Cartesian to Polar1/2 -> Polar to Cartesian/2
  Mux/1 -> Demux1/1
  Idq_gc/1 -> Demux/1
  w/1 -> [w]
  Constant2/1 -> Product1/2
  Discrete PI Controller1/1 -> Demux3/1
  Mux2/1 -> Discrete PI Controller1/1
  Demux2/1 -> Sum3/1  "Vd"
  Constant1/1 -> Product/1
  Vdqs/1 -> Demux2/1
  Demux/2 -> Sum2/1  "Iq"
  Demux/1 -> Sum4/2  "Id"
  Product/1 -> Sum3/2
  Constant3/1 -> Product2/1
  Constant4/1 -> Product3/2
  Product1/1 -> Sum5/2
  Demux2/2 -> Sum5/3  "Vq"
  Product2/1 -> Sum3/3
  Product3/1 -> Sum5/1
  Sum4/1 -> Mux2/1
  Sum2/1 -> Mux2/2
  [w] -> Product1/3
  [w] -> Product/2
  [iq_ref] -> Product/3
  [id_ref] -> Product2/2
  [iq_ref] -> Product3/1
  [id_ref] -> Product1/1
  Demux3/1 -> Sum1/2  "vd'"
  Demux3/2 -> Sum6/1  "vq'"
  Demux1/2 -> [iq_ref], Sum2/2  "Iq_ref"
  Demux1/1 -> Sum4/1, [id_ref]  "Id_ref"
  Sum3/1 -> Sum1/1
  Sum5/1 -> Sum6/2
  Discrete PI Controller/1 -> Mux/1  "Id_ref"
  Sum7/1 -> ->pu/1
  ->pu/1 -> Discrete PI Controller/1
  Vdc/1 -> [Vdc], Sum7/2
  Iq_ref/1 -> Mux/2  "Iq_ref"
  Vdc_ref (V)/1 -> Sum7/1
